simulink model "gain_scheduling_sm_1_gain_scheduling_WP5_seno_frequenza_1"  (R2023b)
settings: Solver=VariableStepAuto  StartTime=0.0  StopTime=50  RelTol=1e-3
values from neighbouring files (symbols this model uses):
  omega_n = 2.63/Tr    (= 9.74074074074)    [gain_sheduling_WP5.m]
  zita = input(2)    [GS_compute_gains_PP.m]    (also in compute_gains_WP5.m; gain_sheduling_WP5.m = 0.95)
settings Model: Creator=miche  LastModifiedBy=miche

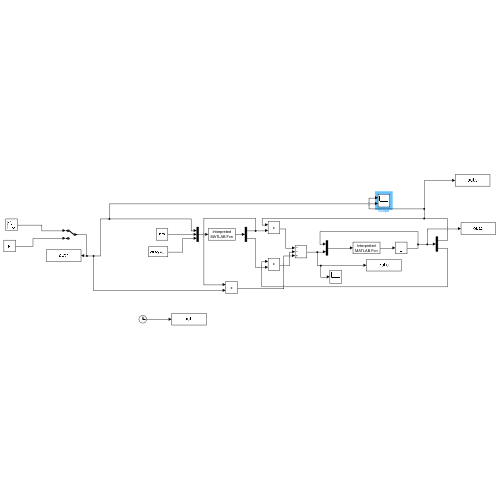
[thumbnail: Simulink's stored preview of the top-level diagram]
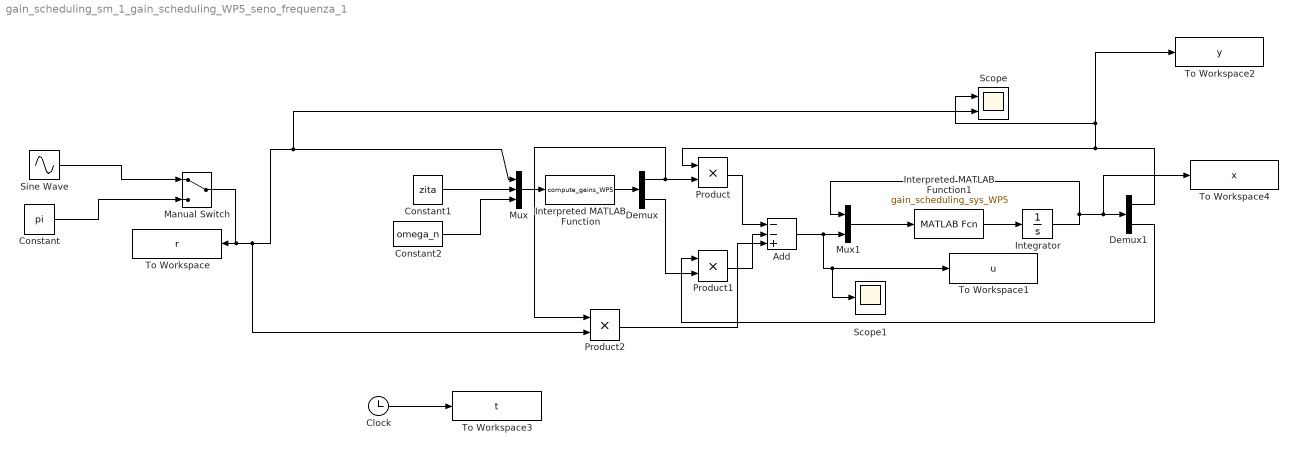
== system gain_scheduling_sm_1_gain_scheduling_WP5_seno_frequenza_1 ==
  Add : Sum  Inputs=--+
  Clock : Clock
  Constant : Constant  Value=pi
  Constant1 : Constant  Value=zita
  Constant2 : Constant  Value=omega_n
  Demux : Demux  Outputs=2
  Demux1 : Demux  Outputs=2
  Integrator : Integrator
  Interpreted MATLAB Function : MATLABFcn  MATLABFcn=compute_gains_WP5  OutputDimensions=2
  Interpreted MATLAB Function1 : MATLABFcn  MATLABFcn=gain_scheduling_sys_WP5  OutputDimensions=2
  Manual Switch : ManualSwitch
  Mux : Mux  Inputs=3
  Mux1 : Mux  Inputs=2
  Product : Product
  Product1 : Product
  Product2 : Product
  Scope : Scope  NumInputPorts=2
  Scope1 : Scope
  Sine Wave : Sin  Amplitude=3.14  SampleTime=0
  To Workspace : ToWorkspace  VariableName=r  SampleTime=-1
  To Workspace1 : ToWorkspace  VariableName=u  SampleTime=-1
  To Workspace2 : ToWorkspace  VariableName=y  SampleTime=-1
  To Workspace3 : ToWorkspace  VariableName=t  SampleTime=-1
  To Workspace4 : ToWorkspace  VariableName=x  SampleTime=-1
  wires:
  Mux/1 -> Interpreted MATLAB Function/1
  Interpreted MATLAB Function/1 -> Demux/1
  Constant/1 -> Manual Switch/2
  Manual Switch/1 -> Product2/2, Scope/2, Mux/1, To Workspace/1
  Mux1/1 -> Interpreted MATLAB Function1/1
  Interpreted MATLAB Function1/1 -> Integrator/1
  Integrator/1 -> To Workspace4/1, Demux1/1, Mux1/1
  Product/1 -> Add/1
  Product1/1 -> Add/2
  Add/1 -> Scope1/1, To Workspace1/1, Mux1/2
  Demux/1 -> Product2/1, Product/2
  Demux/2 -> Product1/2
  Constant1/1 -> Mux/2
  Constant2/1 -> Mux/3
  Demux1/1 -> Product/1, To Workspace2/1, Scope/1
  Sine Wave/1 -> Manual Switch/1
  Demux1/2 -> Product1/1
  Product2/1 -> Add/3
  Clock/1 -> To Workspace3/1
